simulink model "Guidance_Model_Param_StatesRep_Workspace"  (R2024b)
settings: Solver=VariableStepAuto  StartTime=0.0  StopTime=10.0  RelTol=1e-3
undefined symbols (not defined in the file): Pitch, Roll, Thrust, YawRate
libraries: uavalgslib x1
settings Model: Creator=Adi  LastModifiedBy=Adi

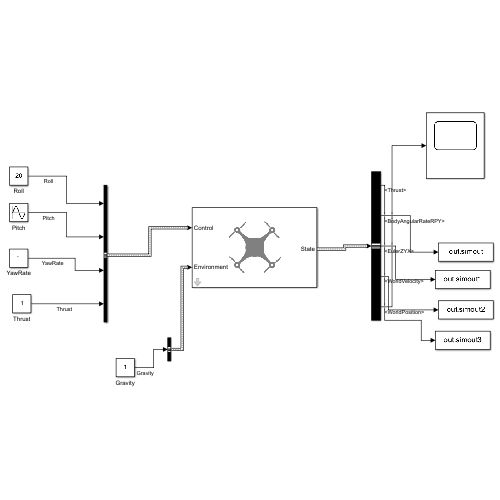
[thumbnail: Simulink's stored preview of the top-level diagram]
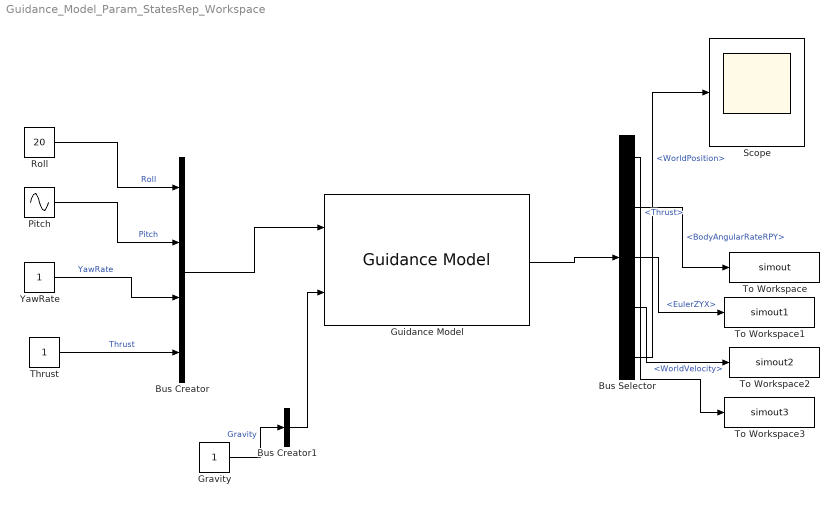
== system Guidance_Model_Param_StatesRep_Workspace ==
  Bus Creator : BusCreator  Inputs=Roll,Pitch,YawRate,Thrust  OutDataTypeStr=Bus: MultirotorGuidanceControlBus  NonVirtualBus=on
  Bus Creator1 : BusCreator  Inputs=Gravity  OutDataTypeStr=Bus: MultirotorGuidanceEnvironmentBus  NonVirtualBus=on
  Bus Selector : BusSelector  OutputSignals=Thrust,BodyAngularRateRPY,EulerZYX,WorldVelocity,WorldPosition
  Gravity : Constant
  Guidance Model : uavalgslib/Guidance Model  ModelType=MultirotorGuidance  SpecifiedDataType=double  SimulateUsing=Interpreted execution  InitialWorldPositionMultirotor=[0; 0; 0]  InitialWorldVelocityMultirotor=[0; 0; 0]  InitialEulerZYXMultirotor=[0; 0; 0]  InitialBodyAngularRateRPYMultirotor=[0; 0; 0]  InitialThrustMultirotor=0  InitialNorthFixedWing=0  InitialEastFixedWing=0  InitialHeightFixedWing=0  InitialAirSpeedFixedWing=0  InitialHeadingAngleFixedWing=0  InitialFlightPathAngleFixedWing=0  InitialRollAngleFixedWing=0  InitialRollAngleRateFixedWing=0  PDRollMultirotor=[3402.97,116.67]  PDPitchMultirotor=[3402.97, 116.67]  PYawRateMultirotor=1950  PThrustMultirotor=3900  MassMultirotor=0.1  PHeightFixedWing=3.9  PHeadingAngleFixedWing=3.9  PFlightPathAngleFixedWing=39  PDRollFixedWing=[3402.97, 116.67]  PAirSpeedFixedWing=1  FlightPathAngleLimitsFixedWing=[-pi/2, pi/2]  StateBusName='MultirotorGuidanceStateBus'  ControlBusName='MultirotorGuidanceControlBus'  EnvironmentBusName='MultirotorGuidanceEnvironmentBus'  DataType=double
  Pitch : Sin  SampleTime=0
  Roll : Constant  Value=20
  Scope : Scope
  Thrust : Constant
  To Workspace : ToWorkspace  VariableName=simout  SaveFormat=Timeseries  SampleTime=-1
      settings: Decimation=4
  To Workspace1 : ToWorkspace  VariableName=simout1  SaveFormat=Timeseries  SampleTime=-1
  To Workspace2 : ToWorkspace  VariableName=simout2  SaveFormat=Timeseries  SampleTime=-1
  To Workspace3 : ToWorkspace  VariableName=simout3  SaveFormat=Timeseries  SampleTime=-1
  YawRate : Constant
  wires:
  Gravity/1 -> Bus Creator1/1  "Gravity"
  Bus Creator1/1 -> Guidance Model/2
  Thrust/1 -> Bus Creator/4  "Thrust"
  YawRate/1 -> Bus Creator/3  "YawRate"
  Roll/1 -> Bus Creator/1  "Roll"
  Pitch/1 -> Bus Creator/2  "Pitch"
  Bus Creator/1 -> Guidance Model/1
  Guidance Model/1 -> Bus Selector/1
  Bus Selector/1 -> To Workspace3/1  "<Thrust>"
  Bus Selector/2 -> To Workspace/1  "<BodyAngularRateRPY>"
  Bus Selector/3 -> To Workspace1/1  "<EulerZYX>"
  Bus Selector/4 -> To Workspace2/1  "<WorldVelocity>"
  Bus Selector/5 -> Scope/1  "<WorldPosition>"
